simulink model "CoffeeReactor_ex2_ver2018"  (R2018a)
settings: Solver=ode4  StartTime=0.0  StopTime=simulationParameters.Tsim  FixedStep=simulationParameters.Tint  RelTol=1e-3
undefined symbols (not defined in the file): flagLinear, ReactorModel_StateUpdate, simulationParameters
settings Model: Creator=simone  LastModifiedBy=fabiomosele
settings DataIOCC: SaveOutput=off  SignalLogging=off  DSMLogging=off  SaveTime=off
settings SFSimCC: SimUseLocalCustomCode=on
settings RTWCC: RTWUseLocalCustomCode=on

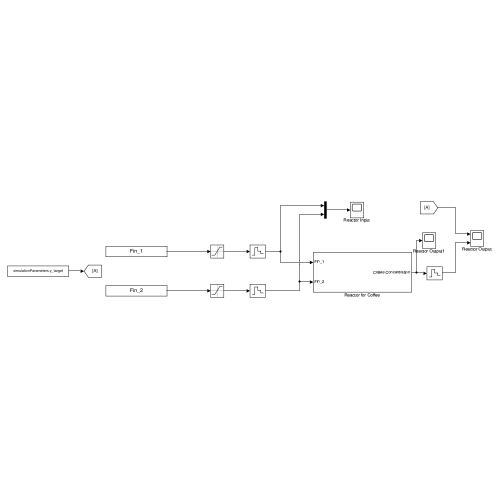
[thumbnail: Simulink's stored preview of the top-level diagram]
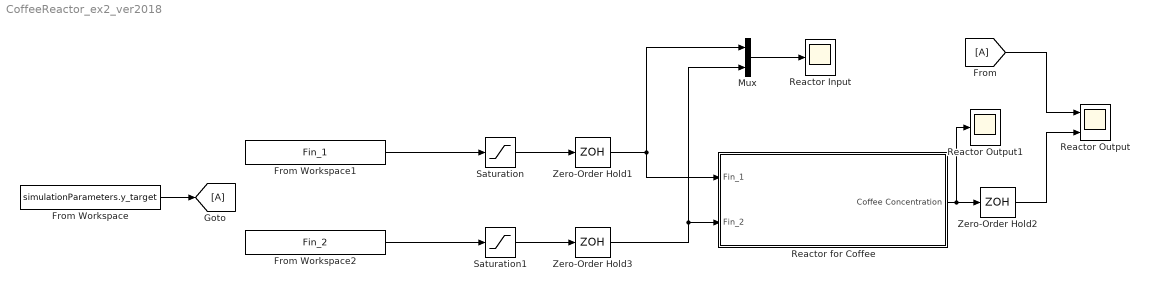
== system CoffeeReactor_ex2_ver2018 ==
  From Workspace : FromWorkspace  VariableName=simulationParameters.y_target  OutputAfterFinalValue=Holding final value
  From Workspace1 : FromWorkspace  VariableName=Fin_1  OutputAfterFinalValue=Holding final value
  From Workspace2 : FromWorkspace  VariableName=Fin_2  OutputAfterFinalValue=Holding final value
  Mux : Mux  Inputs=2
  Reactor Input : Scope
  Reactor Output : Scope  NumInputPorts=2
  Reactor Output1 : Scope
  Reactor for Coffee : Subsystem
  Saturation : Saturate  UpperLimit=simulationParameters.Fin1_max  LowerLimit=simulationParameters.Fin1_min
  Saturation1 : Saturate  UpperLimit=simulationParameters.Fin2_max  LowerLimit=simulationParameters.Fin2_min
  Zero-Order Hold1 : ZeroOrderHold  SampleTime=simulationParameters.Ts
  Zero-Order Hold2 : ZeroOrderHold  SampleTime=simulationParameters.Ts
  Zero-Order Hold3 : ZeroOrderHold  SampleTime=simulationParameters.Ts
  wires:
  Reactor for Coffee/1(Coffee Concentration) -> Zero-Order Hold2/1, Reactor Output1/1
  Zero-Order Hold2/1 -> Reactor Output/2
  [A] -> Reactor Output/1
  Mux/1 -> Reactor Input/1
  From Workspace2/1 -> Saturation1/1
  From Workspace1/1 -> Saturation/1
  Zero-Order Hold1/1 -> Reactor for Coffee/1(Fin_1), Mux/1
  Zero-Order Hold3/1 -> Reactor for Coffee/2(Fin_2), Mux/2
  Saturation/1 -> Zero-Order Hold1/1
  Saturation1/1 -> Zero-Order Hold3/1
  From Workspace/1 -> [A]

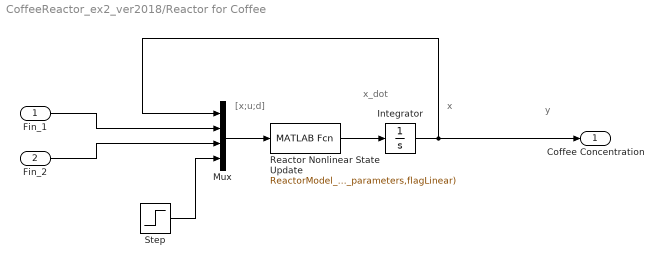
== system CoffeeReactor_ex2_ver2018/Reactor for Coffee ==
  note: y
  note: [x;u;d]
  note: x
  note: x_dot
  Fin_1 : Inport
  Fin_2 : Inport  Port=2
  Integrator : Integrator  InitialCondition=simulationParameters.Reactor_parameters.x_0
  Mux : Mux
  Reactor Nonlinear State Update : MATLABFcn  MATLABFcn=ReactorModel_StateUpdate(u(1),u(2:3),u(4),simulationParameters.Reactor_parameters,flagLinear)  OutputDimensions=simulationParameters.Reactor_parameters.n
  Step : Step  Time=simulationParameters.Reactor_parameters.Tdist  After=simulationParameters.Reactor_parameters.Adist  SampleTime=0
  Coffee Concentration : Outport
  wires:
  Mux/1 -> Reactor Nonlinear State Update/1
  Fin_2/1 -> Mux/3
  Reactor Nonlinear State Update/1 -> Integrator/1
  Fin_1/1 -> Mux/2
  Integrator/1 -> Mux/1, Coffee Concentration/1
  Step/1 -> Mux/4
